simulink library "Driver_Long_Lat_Stanley"  (R2020b)
settings: Solver=VariableStepAuto  StartTime=0.0  StopTime=10.0  RelTol=1e-3
undefined symbols (not defined in the file): Driver
libraries: autolibutils x2, simulink x2, autolibsharedcommon x2, drivingvehiclecontroller x1, Maneuver_Get_Pose x1
(part 2 of 2)

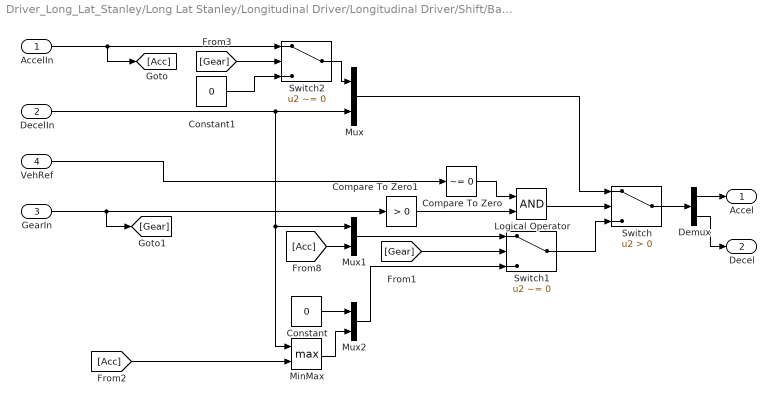
== system Driver_Long_Lat_Stanley/Long Lat Stanley/Longitudinal Driver/Longitudinal Driver/Shift/Basic/Reverse Change ==
  AccelIn : Inport
  DecelIn : Inport  Port=2
  GearIn : Inport  Port=3
  VehRef : Inport  Port=4
  Compare To Zero : simulink/Logic and Bit Operations/Compare To Zero  relop=~=  OutDataTypeStr=boolean  ZeroCross=off
  Compare To Zero1 : simulink/Logic and Bit Operations/Compare To Zero  relop=>  OutDataTypeStr=boolean
  Constant : Constant  Value=0
  Constant1 : Constant  Value=0
  Demux : Demux  Outputs=2
  Logical Operator : Logic  AllPortsSameDT=off  OutDataTypeStr=boolean
  MinMax : MinMax  Function=max  Inputs=2  ZeroCross=off
  Mux : Mux  Inputs=2
  Mux1 : Mux  Inputs=2
  Mux2 : Mux  Inputs=2
  Switch : Switch  Criteria=u2 > Threshold  ZeroCross=off
  Switch1 : Switch  Criteria=u2 ~= 0  ZeroCross=off
  Switch2 : Switch  Criteria=u2 ~= 0  ZeroCross=off
  Accel : Outport  VectorParamsAs1DForOutWhenUnconnected=off
  Decel : Outport  Port=2  VectorParamsAs1DForOutWhenUnconnected=off
  wires:
  GearIn/1 -> Compare To Zero1/1, [Gear]
  [Gear] -> Switch1/2
  Switch1/1 -> Switch/3
  DecelIn/1 -> Mux1/1, MinMax/1, Mux/2
  Switch/1 -> Demux/1
  MinMax/1 -> Mux2/2
  [Acc] -> MinMax/2
  Demux/1 -> Accel/1
  Demux/2 -> Decel/1
  [Acc] -> Mux1/2
  Mux1/1 -> Switch1/1
  Constant/1 -> Mux2/1
  Mux2/1 -> Switch1/3
  Constant1/1 -> Switch2/3
  AccelIn/1 -> [Acc], Switch2/1
  [Gear] -> Switch2/2
  VehRef/1 -> Compare To Zero/1
  Compare To Zero/1 -> Logical Operator/1
  Mux/1 -> Switch/1
  Logical Operator/1 -> Switch/2
  Compare To Zero1/1 -> Logical Operator/2
  Switch2/1 -> Mux/1

== system Driver_Long_Lat_Stanley/Long Lat Stanley/Longitudinal Driver/Longitudinal Driver/Shift/Scheduled/Shift Controller/calc ==
  note: Determine if next gear will be
      | higher or lower than current gear
  gear : Inport
  pedal : Inport  Port=2
  speed : Inport  Port=3
  f : TriggerPort  TriggerType=function-call  VariantControl=Variant  StatesWhenEnabling=reset
      settings: CopyFcn=Stateflow.SLINSF.SimulinkMan.removeBlockPreDeleteFcn  PreDeleteFcn=Stateflow.SLINSF.SimulinkMan.unsafePredeleteFcn
  Add1 : Sum  Inputs=+-
  Add3 : Sum  Inputs=+-
  Add4 : Sum  Inputs=+-
  Calculate Upshift Threshold : Lookup_n-D  BreakpointsForDimension1=pdlVec  BreakpointsForDimension2=UpGearVec  Table=upShftTbl  ExtrapMethod=Clip  UseLastTableValue=on  InternalRulePriority=Speed  RndMeth=Simplest  InputSameDT=on
      settings: InputPortMap=u0,u1
  Calculate Downshift Threshold : Lookup_n-D  BreakpointsForDimension1=pdlVec  BreakpointsForDimension2=DownGearVec  Table=dwnShftTbl  ExtrapMethod=Clip  UseLastTableValue=on  InternalRulePriority=Speed  RndMeth=Simplest  InputSameDT=on
      settings: InputPortMap=u0,u1
  SpdThr : Outport  VectorParamsAs1DForOutWhenUnconnected=off
  wires:
  pedal/1 -> Calculate Downshift Threshold/1, Calculate Upshift Threshold/1
  gear/1 -> Calculate Downshift Threshold/2, Calculate Upshift Threshold/2
  Calculate Downshift Threshold/1 -> Add3/2
  Calculate Upshift Threshold/1 -> Add1/1
  speed/1 -> Add1/2, Add3/1
  Add1/1 -> Add4/1
  Add3/1 -> Add4/2
  Add4/1 -> SpdThr/1

== system Driver_Long_Lat_Stanley/Long Lat Stanley/Longitudinal Driver/Longitudinal Driver/Shift/Scheduled/Shift Controller/calc_down ==
  gear : Inport
  pedal : Inport  Port=2
  f : TriggerPort  TriggerType=function-call  VariantControl=Variant  StatesWhenEnabling=reset
      settings: CopyFcn=Stateflow.SLINSF.SimulinkMan.removeBlockPreDeleteFcn  PreDeleteFcn=Stateflow.SLINSF.SimulinkMan.unsafePredeleteFcn
  Calculate Downshift Threshold : Lookup_n-D  BreakpointsForDimension1=pdlVec  BreakpointsForDimension2=DownGearVec  Table=dwnShftTbl  ExtrapMethod=Clip  UseLastTableValue=on  InternalRulePriority=Speed  RndMeth=Simplest  InputSameDT=on
      settings: InputPortMap=u0,u1
  down_th : Outport  VectorParamsAs1DForOutWhenUnconnected=off
  wires:
  Calculate Downshift Threshold/1 -> down_th/1
  gear/1 -> Calculate Downshift Threshold/2
  pedal/1 -> Calculate Downshift Threshold/1

== system Driver_Long_Lat_Stanley/Long Lat Stanley/Longitudinal Driver/Longitudinal Driver/Shift/Scheduled/Shift Controller/calc_up ==
  gear : Inport
  pedal : Inport  Port=2
  f : TriggerPort  TriggerType=function-call  VariantControl=Variant  StatesWhenEnabling=reset
      settings: CopyFcn=Stateflow.SLINSF.SimulinkMan.removeBlockPreDeleteFcn  PreDeleteFcn=Stateflow.SLINSF.SimulinkMan.unsafePredeleteFcn
  Calculate Upshift Threshold : Lookup_n-D  BreakpointsForDimension1=pdlVec  BreakpointsForDimension2=UpGearVec  Table=upShftTbl  ExtrapMethod=Clip  UseLastTableValue=on  InternalRulePriority=Speed  RndMeth=Simplest  InputSameDT=on
      settings: InputPortMap=u0,u1
  up_th : Outport  VectorParamsAs1DForOutWhenUnconnected=off
  wires:
  Calculate Upshift Threshold/1 -> up_th/1
  pedal/1 -> Calculate Upshift Threshold/1
  gear/1 -> Calculate Upshift Threshold/2

== system Driver_Long_Lat_Stanley/Long Lat Stanley/Longitudinal Driver/Longitudinal Driver/Control/Mapped/Accel Override/Enabled Subsystem ==
  In1 : Inport
  Enable : EnablePort
  Out1 : Outport
  wires:
  In1/1 -> Out1/1

== system Driver_Long_Lat_Stanley/Long Lat Stanley/Longitudinal Driver/Longitudinal Driver/Control/Mapped/Deccel Override/Enabled Subsystem ==
  In1 : Inport
  Enable : EnablePort
  Out1 : Outport
  wires:
  In1/1 -> Out1/1

== system Driver_Long_Lat_Stanley/Long Lat Stanley/Longitudinal Driver/Longitudinal Driver/Control/Predictive/Accel Override/Enabled Subsystem ==
  In1 : Inport
  Enable : EnablePort
  Out1 : Outport
  wires:
  In1/1 -> Out1/1

== system Driver_Long_Lat_Stanley/Long Lat Stanley/Longitudinal Driver/Longitudinal Driver/Control/Predictive/Deccel Override/Enabled Subsystem ==
  In1 : Inport
  Enable : EnablePort
  Out1 : Outport
  wires:
  In1/1 -> Out1/1

== system Driver_Long_Lat_Stanley/Long Lat Stanley/Longitudinal Driver/Longitudinal Driver/Control/Predictive/Powertrain Response/Filtered ==
  u : Inport
  Constant : Constant  Value=(1/tauPt)*pi*2
  Divide1 : Product  Inputs=**
  Integrator1 : Integrator
  Sum : Sum  Inputs=|+-
  Switch : Switch  Criteria=u2 > Threshold  ZeroCross=off
  u' : Outport  VectorParamsAs1DForOutWhenUnconnected=off
  wires:
  Constant/1 -> Divide1/2
  Sum/1 -> Divide1/1
  Integrator1/1 -> Switch/2, Switch/1
  Switch/1 -> Sum/2, u'/1
  Divide1/1 -> Integrator1/1
  u/1 -> Switch/3, Sum/1

== system Driver_Long_Lat_Stanley/Long Lat Stanley/Longitudinal Driver/Longitudinal Driver/Control/Predictive/Powertrain Response/Unfiltered ==
  u : Inport
  u' : Outport  VectorParamsAs1DForOutWhenUnconnected=off
  wires:
  u/1 -> u'/1

== system Driver_Long_Lat_Stanley/Long Lat Stanley/Longitudinal Driver/Longitudinal Driver/Control/Scalar/Accel Override/Enabled Subsystem ==
  In1 : Inport
  Enable : EnablePort
  Out1 : Outport
  wires:
  In1/1 -> Out1/1

== system Driver_Long_Lat_Stanley/Long Lat Stanley/Longitudinal Driver/Longitudinal Driver/Control/Scalar/Deccel Override/Enabled Subsystem ==
  In1 : Inport
  Enable : EnablePort
  Out1 : Outport
  wires:
  In1/1 -> Out1/1

== matlab function Driver_Long_Lat_Stanley/Long Lat Stanley/Longitudinal Driver/Longitudinal Driver/Control/Predictive/Setup ==
  data: m parameter size=1; U input size=1; F output size=[2,2]; Kpt parameter size=1; G output size=[2,1]; a_star output size=1; b_star output size=[1,2]; Lvv parameter size=1; aR parameter size=1; bR parameter size=1; cR parameter size=1; tau parameter size=1
function [F,G,a_star,b_star] = fcn(m,U,Kpt,Lvv, aR, bR, cR,tau)%#codegen
coder.allowpcode('plain')
% Copyright 2018 The MathWorks, Inc.

[F,G,a_star,b_star] = automlvehdynlongdriversetup(aR,bR,cR,m,Kpt,Lvv,U,tau);
end

== matlab function Driver_Long_Lat_Stanley/Long Lat Stanley/Longitudinal Driver/Longitudinal Driver/Control/Predictive/Vehicle ==
  data: F input; G input; u input; x output size=[2 1]; x_o input
function x = fcn(F,G,u,x_o) %#codegen
coder.allowpcode('plain')
% Copyright 20178 The MathWorks, Inc.
x = automlvehdynlongdriverplant(F,G,u,x_o);
end

== stateflow chart Driver_Long_Lat_Stanley/Long Lat Stanley/Longitudinal Driver/Longitudinal Driver/Shift/Basic/Shift Controller ==
  settings: sampleTime=0.01
  state GearSelect [parallel]
    settings: executionOrder=1
    state Reverse
      entry:
      Gear = -1;
    state Neutral
      entry:
      Gear = 0;
    state Odd
      en:Gear = GearState;
    (default) -> (junction 472) : /* InitialGear */
        | {Gear = GearInit;
        | GearState=GearInit;}
    (junction 472) -> (junction 474) [order 1] : [GearInit<0]
    (junction 474) -> Reverse
    (junction 472) -> (junction 487) [order 2]
    (junction 487) -> (junction 475) [order 1] : [GearInit==0]
    (junction 487) -> (junction 473) [order 2]
    (junction 475) -> Neutral
    (junction 473) -> Odd
    Neutral -> Reverse [order 2] : after(tShift,sec)
        | [VehRef<0]
        | {GearState=GearState-1;}
    Neutral -> Odd [order 1] : after(tShift,sec)
        | [VehRef>0 &&pedal>0]
        | {GearState=GearState+1;}
    Reverse -> Neutral : after(tShift,sec)
        | [VehRef>=0]
        | {GearState=GearState+1;}
    Odd -> Neutral : after(tShift,sec)
        | [(Brake>=0&&speed<=0&&pedal<=0)||VehRef<=0]
        | {GearState=GearState-1;}
  data: pedal input; Brake input; VehRef input; Gear output double; GearState local double size=1 =GearInit; tShift parameter double; GearInit parameter double; speed input

== stateflow chart Driver_Long_Lat_Stanley/Long Lat Stanley/Longitudinal Driver/Longitudinal Driver/Shift/Scheduled/Shift Controller ==
  settings: sampleTime=0.01
  state GearSelect [parallel]
    settings: executionOrder=1
    state Reverse
      entry:
      GearState = -1;
    state Neutral
      entry:
      GearState = 0;
    state Odd
      en:GearState = Gear;
      du:[SpdThr]=calc(Gear,pedal,speed);
    state Even
      en:GearState = Gear;
      du:[SpdThr]=calc(Gear,pedal,speed);
    state Park
      entry:
      GearState = 80;
    (default) -> (junction 461) : /* InitialGear */
        | {Gear = GearInit;}
    (junction 461) -> (junction 463) [order 1] : [GearInit==80]
    (junction 463) -> Park
    (junction 461) -> (junction 441) [order 2]
    (junction 441) -> (junction 442) [order 1] : [GearInit<0]
    (junction 442) -> Reverse
    (junction 441) -> (junction 457) [order 2]
    (junction 457) -> (junction 459) [order 1] : [GearInit==0]
    (junction 459) -> Neutral
    (junction 457) -> (junction 445) [order 2]
    (junction 445) -> (junction 446) [order 1] : [GearInit%%2==0]
    (junction 445) -> Odd [order 2]
    (junction 446) -> Even
    (junction 363) -> (junction 366)
    (junction 366) -> Odd
    Even -> (junction 363) [order 1] : UP
        | {Gear=Gear+1;}
    Neutral -> Reverse [order 2] : DOWN
        | {Gear=Gear-1;}
    Neutral -> Odd [order 1] : UP
        | {Gear=Gear+1;}
    Odd -> Even [order 1] : UP
        | {Gear=Gear+1;}
    Reverse -> Neutral : UP
        | {Gear=Gear+1;}
    Even -> Odd [order 2] : DOWN
        | {Gear=Gear-1;}
    Neutral -> (junction 380) [order 3]
    (junction 379) -> Neutral
    (junction 370) -> Neutral
    Odd -> (junction 361) [order 2] : DOWN
        | {Gear=Gear-1;}
    (junction 357) -> Even
    Even -> (junction 371) [order 3] : [Gear==0]
    (junction 361) -> (junction 357)
    (junction 380) -> Park : after(tPark,sec)
        | [Brake>0.5&&...
        | speed==0&&...
        | VehRef==0]
    Park -> (junction 379) : [VehRef~=0&&pedal>0]
    (junction 371) -> (junction 370)
  state SelectionState [parallel]
    du:[up_th]=calc_up(GearState,pedal);
    du:[down_th]=calc_down(GearState,pedal);
    settings: executionOrder=2
    state SteadyState
      en:
      clutchControl = 0;
    state preDownShifting
      en:clutchControl = 1;
    state preUpShifting
      en:clutchControl = 1;
    state UpShifting
      en:
      GearState = GearState + 0.5;
    state DownShifting
      en:
      GearState = GearState - 0.5;
    (default) -> SteadyState
    SteadyState -> (junction 128) [order 2] : [VehRef>0&& speed > up_th &&...
        | GearState <= N && ...
        | floor(GearState) == GearState]
    SteadyState -> (junction 423) [order 3] : after(tRev,sec)
        | [VehRef<0&&GearState==0]
    (junction 128) -> preUpShifting
    (junction 423) -> preDownShifting
    SteadyState -> (junction 62) [order 1] : [speed < down_th && ...
        | GearState >=1]
    (junction 62) -> preDownShifting
    (junction 168) -> SteadyState
    (junction 23) -> SteadyState
    (junction 161) -> SteadyState
    preDownShifting -> (junction 168) [order 2] : [speed >= down_th]
    preUpShifting -> (junction 161) [order 2] : [speed <= up_th]
    preUpShifting -> UpShifting [order 1] : after(tClutch,sec)
        | [speed>up_th]
    preDownShifting -> DownShifting [order 1] : after(tClutch, sec)
        | [(speed < down_th - 2) || speed<=0]
    DownShifting -> (junction 23) : {GearSelect.DOWN;}
    UpShifting -> (junction 23) : {GearSelect.UP;}
  state up_th = calc_up(gear,pedal) [function]
  state down_th = calc_down(gear,pedal) [function]
  state SpdThr = calc(gear,pedal,speed) [function]
  data: gear function_input; pedal function_input; up_th function_output; gear function_input; pedal function_input; down_th function_output; gear function_input; pedal function_input; SpdThr function_output; speed function_input; Gear output double =GearInit; clutchControl output double; pedal input; Brake input; VehRef input; speed input; SpdThr local double; up_th local double; down_th local double; tPark parameter; tRev parameter; GearInit parameter double; N local double =size(upShftTbl,2); tClutch parameter; GearState local double
  events: DOWN local EITHER_EDGE_EVENT; UP local EITHER_EDGE_EVENT
